simulink model "PMSM_foc_mod"  (R2020a)
settings: Solver=ode45  StartTime=0.0  StopTime=.5  MaxStep=1e-3  RelTol=1e-3
InitFcn:
  | %Rs = 2.98;
  | %phi_mg = .125;
  | %Jm = .47/10000;
  | %Bv = 1.1/10000;
  | %Zp = 2;
  | %Ld = 7/1000;
  | %Lq = 7/1000;
  | %Tl = 0;
  | 
  | Rs = 4.3;
  | phi_mg = .272;
  | Jm = .000179;
  | Bv = 1.1/10000;
  | Zp = 4;
  | Ld = 67e-3;
  | Lq = 67e-3;
  | Tl = 0;
  | 
  | Vdc = 220*2*sqrt(2);
libraries: powerlib x17, simulink x6, dspsigops x3, powerlib_meascontrol x3
settings Model: Creator=TELE  LastModifiedBy=TELE
settings DataIOCC: ReturnWorkspaceOutputs=off
settings DebuggingCC: ArithmeticOperatorsInVariantConditions=warning
settings SFSimCC: SimUseLocalCustomCode=off  CustomCodeUndefinedFunction=UseInterfaceOnly
settings RTWCC: RTWUseLocalCustomCode=off

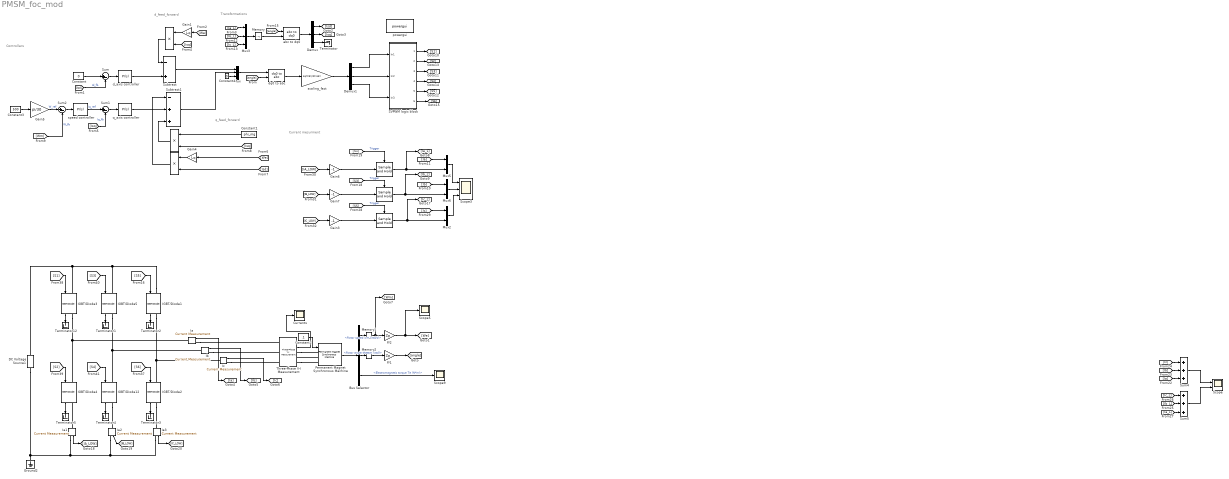
== system PMSM_foc_mod ==
  note: Controllers
  note: Transformations
  note: Current mesurment
  note: d_feed_forward
  note: q_feed_forward
  "  " : dspsigops/Sample and Hold  trig=Rising edge  initCond=0  latchinput=off
  "     " : dspsigops/Sample and Hold  trig=Rising edge  initCond=0  latchinput=off
  "         " : Product
  "           " : Product
  "                         " : Product
  "                                " : dspsigops/Sample and Hold  trig=Rising edge  initCond=0  latchinput=off
  Bus Selector : BusSelector  OutputSignals=Rotor speed wm (rad/s),Rotor angle thetam (rad),Electromagnetic torque Te (N*m)
  Constant : Constant  Value=0
  Constant1 : Constant  Value=phi_mg
  Constant2 : Constant  Value=.1
  Constant3 : Constant  Value=500
  Constant4 : Constant  Value=0
  Currents : Scope
  DC Voltage Source1 : powerlib/Electrical Sources/DC Voltage Source  Amplitude=Vdc  Measurements=None
  Demux : Demux  Outputs=3
  Demux1 : Demux  Outputs=3
  Gain1 : Gain  Gain=Lq
  Gain3 : Gain  Gain=-1
  Gain4 : Gain  Gain=Lq
  Gain5 : Gain  Gain=pi/30
  Gain6 : Gain  Gain=-1
  Gain7 : Gain  Gain=-1
  Ground2 : powerlib/Elements/Ground  LConnTagsString=a
  IGBT/Diode{1..5,12} (6 alike) : powerlib/Power Electronics/IGBT//Diode  Ron=1e-3  Rs=1e5  Cs=inf  Measurements=on
  Ia{,1..3} (4 alike) : powerlib/Measurements/Current Measurement  PhasorSimulation=off  OutputType=Complex  PSBequivalent=0
  Ib : powerlib/Measurements/Current Measurement  PhasorSimulation=off  OutputType=Complex  PSBequivalent=0
  Ic : powerlib/Measurements/Current Measurement  PhasorSimulation=off  OutputType=Complex  PSBequivalent=0
  Memory : Memory
  Memory1 : Memory
  Memory2 : Memory
  Mux : Mux  Inputs=3
  Mux2 : Mux  Inputs=2
  Mux3 : Mux  Inputs=3
  Mux5 : Mux  Inputs=2
  Mux6 : Mux  Inputs=2
  P/1 : Gain  Gain=Zp
  P/2 : Gain  Gain=Zp
  Permanent Magnet Synchronous Machine : powerlib/Machines/Permanent Magnet Synchronous Machine  NbPhases=3  FluxDistribution=Sinusoidal  RotorType=Round  MechanicalLoad=Torque Tm  PresetModel=No  ShowDetailedParameters=on  MeasurementBus=off  Resistance=Rs  Inductance=8.5e-3  dqInductances=[8.5e-3,8.5e-3]  La=Ld  MachineConstant=Flux linkage established by magnets (V.s)  Flux=phi_mg  VoltageCst=197.3414  TorqueCst=1.632  Flat=120  Mechanical=[Jm Bv Zp 0]  PolePairs=4  InitialConditions=[0,0, 0,0]  InitialConditions5ph=[0 0 0 0 0 0]  RefAngle=90 degrees behind phase A axis (modified Park)  IterativeDiscreteModel=Trapezoidal non iterative  TsBlock=-1  TsPowergui=0
  SVPWM logic block : Subsystem
  Scope : Scope  NumInputPorts=2
  Scope3 : Scope  NumInputPorts=3
  Scope5 : Scope
  Scope9 : Scope
  Subtract : Sum  Inputs=-+
  Subtract1 : Sum  Inputs=-++
  Sum : Sum  Inputs=|+-
  Sum1 : Sum  Inputs=|+-
  Sum2 : Sum  Inputs=|+-
  Sum4 : Sum  Inputs=+++
  Sum5 : Sum  Inputs=+++
  Terminator{,1..5,12} (7 alike) : Terminator
  Three-Phase V-I Measurement : powerlib/Measurements/Three-Phase V-I Measurement  VoltageMeasurement=phase-to-ground  SetLabelV=off  LabelV=Vabc  Vpu=off  VpuLL=off  CurrentMeasurement=yes  SetLabelI=off  LabelI=Iabc  Ipu=off  Pbase=100e6  Vbase=500e3  OutputType=Complex  PhasorSimulation=off  PSBequivalent=0
  abc to dq0 : powerlib_meascontrol/Transformations/abc to dq0  Alignment=90 degrees behind phase A axis
  d_axis controller : simulink/Continuous/PID Controller  Controller=PI  Form=Parallel  TimeDomain=Continuous-time  UseExternalTs=off  SampleTime=-1  IntegratorMethod=Forward Euler  FilterMethod=Forward Euler  ControllerParametersSource=internal  P=190.322068059803  I=236063.180042371  D=0  UseFilter=on  N=100  TunerSelectOption=Transfer Function Based (PID Tuner App)  InitialConditionSource=internal  InitialConditionForIntegrator=0  InitialConditionForFilter=0  DifferentiatorICPrevScaledInput=0  ExternalReset=none  TrackingMode=off  Kt=1  LimitOutput=off  UpperSaturationLimit=inf  LowerSaturationLimit=-inf  LinearizeAsGain=on  AntiWindupMode=none  Kb=1  POutMin=[]  POutMax=[]  IOutMin=[]  IOutMax=[]  DOutMin=[]  DOutMax=[]  NOutMin=[]  NOutMax=[]  SumOutMin=[]  SumOutMax=[]  SaturationOutMin=[]  SaturationOutMax=[]  PParamMin=[]  PParamMax=[]  IParamMin=[]  IParamMax=[]  DParamMin=[]  DParamMax=[]  NParamMin=[]  NParamMax=[]  KbParamMin=[]  KbParamMax=[]  KtParamMin=[]  KtParamMax=[]  KbOutMin=[]  KbOutMax=[]  KtOutMin=[]  KtOutMax=[]  IntegratorOutMin=[]  IntegratorOutMax=[]  FilterOutMin=[]  FilterOutMax=[]  SumI1OutMin=[]  SumI1OutMax=[]  SumI2OutMin=[]  SumI2OutMax=[]  SumI3OutMin=[]  SumI3OutMax=[]  SumI4OutMin=[]  SumI4OutMax=[]  SumDOutMin=[]  SumDOutMax=[]  DifferentiatorOutMin=[]  DifferentiatorOutMax=[]  FilterDiffOutCoefMin=[]  FilterDiffOutCoefMax=[]  ReciprocalOutMin=[]  ReciprocalOutMax=[]  SumDenOutMin=[]  SumDenOutMax=[]  SumNumOutMin=[]  SumNumOutMax=[]  DivideOutMin=[]  DivideOutMax=[]  UdiffTsProdOutMin=[]  UdiffTsProdOutMax=[]  NTsProdOutMin=[]  NTsProdOutMax=[]  UintegralTsProdOutMin=[]  UintegralTsProdOutMax=[]  UngainTsProdOutMin=[]  UngainTsProdOutMax=[]  IntegratorContinuousStateAttributes=''  IntegratorStateMustResolveToSignalObject=off  IntegratorRTWStateStorageClass=Auto  FilterContinuousStateAttributes=''  FilterStateMustResolveToSignalObject=off  FilterRTWStateStorageClass=Auto  ParallelPVariant=InternalParameters  IdealPVariant=Disabled  IVariant=InternalParameters  DVariant=Disabled  IntegratorVariant=Continuous  SatVariant=Disabled  AWVariant=Passthrough  PCopyVariant=Disabled  TRVariant=Disabled  FdbkBlocksVariant=Forward  IdealPFdbkVariant=Disabled  SatFdbkVariant=Disabled  DerivativeFilterVariant=Disabled  NVariant=Disabled  NCopyVariant=Disabled_SignalSpec  FilterICVariant=Disabled  IntegratorICVariant=InternalICs  ExternalResetVariant=Disabled  TRSumVariant=Passthrough  SumFdbkVariant=Disabled  SumVariant=Sum_PI  TsampFilterVariant=InternalTs  TsampNgainVariant=Passthrough  TsampIntegralVariant=Passthrough
  dq0 to abc : powerlib_meascontrol/Transformations/dq0 to abc  Alignment=90 degrees behind phase A axis
  powergui : powerlib/powergui  Priority=1  SimulationMode=Continuous  SampleTime=50e-6  frequency=60  Iterations=50  frequencyindice=0  Pbase=100e6  ErrMax=1e-4  UnitsV=kV  UnitsW=MW  buscounter=0  FunctionMessages=off  echomessages=off  EnableUseOfTLC=off  CurrentSourceSwitches=off  DisableSnubberDevices=off  DisableRonSwitches=off  DisableVfSwitches=off  DisplayEquations=off  AutomaticDiscreteSolvers=off  SolverType=Tustin/Backward Euler (TBE)  Interpol=off  ExternalGateDelay=off  methode=off  Ts=100  x0status=blocks  SPID=on  SwTol=0  HookPort=off  NonlinearTolerance=1e-4  nMaxIteration=100  ContinueOnMaxIteration=off  RestoreLinks=warning  ResistiveCurrentMeasurement=off  Frange=[0:2:500]  Ylog=off  Xlog=on  ShowGrid=off  save=off  variable=ZData  structure=0  ZoomFFT=off  StartTime=0.0  cycles=1  DisplayStyle=1  fundamental=60  FreqAxis=off  MaxFrequency=1000  frequencyindicesteady=1  RmsSteady=1  display=off
  q_axis controller : simulink/Continuous/PID Controller  Controller=PI  Form=Parallel  TimeDomain=Continuous-time  UseExternalTs=off  SampleTime=-1  IntegratorMethod=Forward Euler  FilterMethod=Forward Euler  ControllerParametersSource=internal  P=190.322068059803  I=236063.180042371  D=0  UseFilter=on  N=100  TunerSelectOption=Transfer Function Based (PID Tuner App)  InitialConditionSource=internal  InitialConditionForIntegrator=0  InitialConditionForFilter=0  DifferentiatorICPrevScaledInput=0  ExternalReset=none  TrackingMode=off  Kt=1  LimitOutput=off  UpperSaturationLimit=inf  LowerSaturationLimit=-inf  LinearizeAsGain=on  AntiWindupMode=none  Kb=1  POutMin=[]  POutMax=[]  IOutMin=[]  IOutMax=[]  DOutMin=[]  DOutMax=[]  NOutMin=[]  NOutMax=[]  SumOutMin=[]  SumOutMax=[]  SaturationOutMin=[]  SaturationOutMax=[]  PParamMin=[]  PParamMax=[]  IParamMin=[]  IParamMax=[]  DParamMin=[]  DParamMax=[]  NParamMin=[]  NParamMax=[]  KbParamMin=[]  KbParamMax=[]  KtParamMin=[]  KtParamMax=[]  KbOutMin=[]  KbOutMax=[]  KtOutMin=[]  KtOutMax=[]  IntegratorOutMin=[]  IntegratorOutMax=[]  FilterOutMin=[]  FilterOutMax=[]  SumI1OutMin=[]  SumI1OutMax=[]  SumI2OutMin=[]  SumI2OutMax=[]  SumI3OutMin=[]  SumI3OutMax=[]  SumI4OutMin=[]  SumI4OutMax=[]  SumDOutMin=[]  SumDOutMax=[]  DifferentiatorOutMin=[]  DifferentiatorOutMax=[]  FilterDiffOutCoefMin=[]  FilterDiffOutCoefMax=[]  ReciprocalOutMin=[]  ReciprocalOutMax=[]  SumDenOutMin=[]  SumDenOutMax=[]  SumNumOutMin=[]  SumNumOutMax=[]  DivideOutMin=[]  DivideOutMax=[]  UdiffTsProdOutMin=[]  UdiffTsProdOutMax=[]  NTsProdOutMin=[]  NTsProdOutMax=[]  UintegralTsProdOutMin=[]  UintegralTsProdOutMax=[]  UngainTsProdOutMin=[]  UngainTsProdOutMax=[]  IntegratorContinuousStateAttributes=''  IntegratorStateMustResolveToSignalObject=off  IntegratorRTWStateStorageClass=Auto  FilterContinuousStateAttributes=''  FilterStateMustResolveToSignalObject=off  FilterRTWStateStorageClass=Auto  ParallelPVariant=InternalParameters  IdealPVariant=Disabled  IVariant=InternalParameters  DVariant=Disabled  IntegratorVariant=Continuous  SatVariant=Disabled  AWVariant=Passthrough  PCopyVariant=Disabled  TRVariant=Disabled  FdbkBlocksVariant=Forward  IdealPFdbkVariant=Disabled  SatFdbkVariant=Disabled  DerivativeFilterVariant=Disabled  NVariant=Disabled  NCopyVariant=Disabled_SignalSpec  FilterICVariant=Disabled  IntegratorICVariant=InternalICs  ExternalResetVariant=Disabled  TRSumVariant=Passthrough  SumFdbkVariant=Disabled  SumVariant=Sum_PI  TsampFilterVariant=InternalTs  TsampNgainVariant=Passthrough  TsampIntegralVariant=Passthrough
  scaling_fact : Gain  Gain=sqrt(3)/(2*Vdc)
  speed controller : simulink/Continuous/PID Controller  Controller=PI  Form=Parallel  TimeDomain=Continuous-time  UseExternalTs=off  SampleTime=-1  IntegratorMethod=Forward Euler  FilterMethod=Forward Euler  ControllerParametersSource=internal  P=0.003810758400944  I=0.0139378856974398  D=0  UseFilter=on  N=100  TunerSelectOption=Transfer Function Based (PID Tuner App)  InitialConditionSource=internal  InitialConditionForIntegrator=0  InitialConditionForFilter=0  DifferentiatorICPrevScaledInput=0  ExternalReset=none  TrackingMode=off  Kt=1  LimitOutput=off  UpperSaturationLimit=inf  LowerSaturationLimit=-inf  LinearizeAsGain=on  AntiWindupMode=none  Kb=1  POutMin=[]  POutMax=[]  IOutMin=[]  IOutMax=[]  DOutMin=[]  DOutMax=[]  NOutMin=[]  NOutMax=[]  SumOutMin=[]  SumOutMax=[]  SaturationOutMin=[]  SaturationOutMax=[]  PParamMin=[]  PParamMax=[]  IParamMin=[]  IParamMax=[]  DParamMin=[]  DParamMax=[]  NParamMin=[]  NParamMax=[]  KbParamMin=[]  KbParamMax=[]  KtParamMin=[]  KtParamMax=[]  KbOutMin=[]  KbOutMax=[]  KtOutMin=[]  KtOutMax=[]  IntegratorOutMin=[]  IntegratorOutMax=[]  FilterOutMin=[]  FilterOutMax=[]  SumI1OutMin=[]  SumI1OutMax=[]  SumI2OutMin=[]  SumI2OutMax=[]  SumI3OutMin=[]  SumI3OutMax=[]  SumI4OutMin=[]  SumI4OutMax=[]  SumDOutMin=[]  SumDOutMax=[]  DifferentiatorOutMin=[]  DifferentiatorOutMax=[]  FilterDiffOutCoefMin=[]  FilterDiffOutCoefMax=[]  ReciprocalOutMin=[]  ReciprocalOutMax=[]  SumDenOutMin=[]  SumDenOutMax=[]  SumNumOutMin=[]  SumNumOutMax=[]  DivideOutMin=[]  DivideOutMax=[]  UdiffTsProdOutMin=[]  UdiffTsProdOutMax=[]  NTsProdOutMin=[]  NTsProdOutMax=[]  UintegralTsProdOutMin=[]  UintegralTsProdOutMax=[]  UngainTsProdOutMin=[]  UngainTsProdOutMax=[]  IntegratorContinuousStateAttributes=''  IntegratorStateMustResolveToSignalObject=off  IntegratorRTWStateStorageClass=Auto  FilterContinuousStateAttributes=''  FilterStateMustResolveToSignalObject=off  FilterRTWStateStorageClass=Auto  ParallelPVariant=InternalParameters  IdealPVariant=Disabled  IVariant=InternalParameters  DVariant=Disabled  IntegratorVariant=Continuous  SatVariant=Disabled  AWVariant=Passthrough  PCopyVariant=Disabled  TRVariant=Disabled  FdbkBlocksVariant=Forward  IdealPFdbkVariant=Disabled  SatFdbkVariant=Disabled  DerivativeFilterVariant=Disabled  NVariant=Disabled  NCopyVariant=Disabled_SignalSpec  FilterICVariant=Disabled  IntegratorICVariant=InternalICs  ExternalResetVariant=Disabled  TRSumVariant=Passthrough  SumFdbkVariant=Disabled  SumVariant=Sum_PI  TsampFilterVariant=InternalTs  TsampNgainVariant=Passthrough  TsampIntegralVariant=Passthrough
  wires:
  Ia/1 -> [Ia]
  Bus Selector/3 -> Scope9/1  "<Electromagnetic torque Te (N*m)>"
  P/2/1 -> Scope5/1, [We]
  Demux1/3 -> SVPWM logic block/3(In3)
  Demux1/2 -> SVPWM logic block/2(In2)
  Demux1/1 -> SVPWM logic block/1(In1)
  scaling_fact/1 -> Demux1/1
  SVPWM logic block/5(5) -> [S5]
  [S4] -> IGBT/Diode12/1
  IGBT/Diode12/1 -> Terminator4/1
  [S5] -> IGBT/Diode1/1
  [S2] -> IGBT/Diode4/1
  SVPWM logic block/3(3) -> [S3]
  [S3] -> IGBT/Diode5/1
  IGBT/Diode2/1 -> Terminator3/1
  IGBT/Diode3/1 -> Terminator12/1
  SVPWM logic block/1(1) -> [S1]
  SVPWM logic block/4(4) -> [S4]
  IGBT/Diode5/1 -> Terminator1/1
  [S1] -> IGBT/Diode3/1
  IGBT/Diode4/1 -> Terminator5/1
  SVPWM logic block/2(2) -> [S2]
  IGBT/Diode1/1 -> Terminator2/1
  [S6] -> IGBT/Diode2/1
  SVPWM logic block/6(6) -> [S6]
  Demux/3 -> Terminator/1
  Demux/2 -> [Isq]
  Demux/1 -> [Isd]
  abc to dq0/1 -> Demux/1
  [angle] -> abc to dq0/2
  Ic/1 -> [Ic]
  Ib/1 -> [Ib]
  [angle] -> dq0 to abc/2
  P/1/1 -> [angle]
  Bus Selector/2 -> Memory2/1  "<Rotor angle thetam (rad)>"
  Mux/1 -> dq0 to abc/1
  Memory1/1 -> [Wm], P/2/1
  Permanent Magnet Synchronous Machine/1 -> Bus Selector/1
  "                         "/1 -> Subtract1/3
  Constant1/1 -> "                         "/1
  [Isq] -> "                         "/2
  q_axis controller/1 -> Subtract1/2
  Sum1/1 -> q_axis controller/1
  [We] -> Gain4/1
  Gain4/1 -> "         "/1
  [Isd] -> "         "/2
  "         "/1 -> Subtract1/1
  Subtract1/1 -> Mux/2
  Subtract/1 -> Mux/1
  "           "/1 -> Subtract/1
  [Isq] -> "           "/2
  Gain1/1 -> "           "/1
  [We] -> Gain1/1
  Sum/1 -> d_axis controller/1
  d_axis controller/1 -> Subtract/2
  speed controller/1 -> Sum1/1  "Iq_ref"
  Sum2/1 -> speed controller/1
  Constant3/1 -> Gain5/1
  Constant2/1 -> Permanent Magnet Synchronous Machine/1
  Constant4/1 -> Mux/3
  Three-Phase V-I Measurement/2 -> Currents/1
  Gain5/1 -> Sum2/1  "W_ref"
  Gain6/1 -> "  "/1
  Gain7/1 -> "     "/1
  "     "/1 -> [Ib_L], Mux6/2
  "  "/1 -> [Ia_L], Mux5/2
  [S3] -> "     "/Trigger  "Trigger"
  Mux5/1 -> Scope3/1
  Mux6/1 -> Scope3/2
  [Ib] -> Mux6/1
  [Ia] -> Mux5/1
  [S1] -> "  "/Trigger  "Trigger"
  Mux3/1 -> Memory/1
  dq0 to abc/1 -> scaling_fact/1
  Constant/1 -> Sum/1
  [Isd] -> Sum/2  "Id_fb"
  [Wm] -> Sum2/2  "W_fb"
  [Isq] -> Sum1/2  "Iq_fb"
  Memory/1 -> abc to dq0/1
  [Ia_L] -> Mux3/1
  [Ic_L] -> Mux3/3
  [Ib_L] -> Mux3/2
  Sum4/1 -> Scope/1
  [Ib] -> Sum4/2
  [Ic] -> Sum4/1
  [Ia] -> Sum4/3
  [Ic_L] -> Sum5/1
  [Ib_L] -> Sum5/2
  [Ia_L] -> Sum5/3
  Sum5/1 -> Scope/2
  [S5] -> "                                "/Trigger  "Trigger"
  Gain3/1 -> "                                "/1
  "                                "/1 -> Mux2/2, [Ic_L]
  [Ic] -> Mux2/1
  Mux2/1 -> Scope3/3
  Bus Selector/1 -> Memory1/1  "<Rotor speed wm (rad/s)>"
  Memory2/1 -> P/1/1
  Ia1/1 -> [IA_LOW]
  Ia2/1 -> [IB_LOW]
  Ia3/1 -> [IC_LOW]
  [IA_LOW] -> Gain6/1
  [IB_LOW] -> Gain7/1
  [IC_LOW] -> Gain3/1
  connections:
  IGBT/Diode1/LConn1 -- IGBT/Diode3/LConn1 -- DC Voltage Source1/RConn1 -- IGBT/Diode5/LConn1
  DC Voltage Source1/LConn1 -- Ground2/LConn1 -- Ia1/RConn1 -- Ia3/RConn1 -- Ia2/RConn1
  IGBT/Diode5/RConn1 -- IGBT/Diode12/LConn1 -- Ib/LConn1
  IGBT/Diode3/RConn1 -- IGBT/Diode4/LConn1 -- Ia/LConn1
  IGBT/Diode1/RConn1 -- Ic/LConn1 -- IGBT/Diode2/LConn1
  Three-Phase V-I Measurement/RConn3 -- Permanent Magnet Synchronous Machine/LConn3
  Permanent Magnet Synchronous Machine/LConn2 -- Three-Phase V-I Measurement/RConn2
  Three-Phase V-I Measurement/RConn1 -- Permanent Magnet Synchronous Machine/LConn1
  Ic/RConn1 -- Three-Phase V-I Measurement/LConn3
  Ib/RConn1 -- Three-Phase V-I Measurement/LConn2
  Ia/RConn1 -- Three-Phase V-I Measurement/LConn1
  Ia1/LConn1 -- IGBT/Diode4/RConn1
  IGBT/Diode12/RConn1 -- Ia2/LConn1
  IGBT/Diode2/RConn1 -- Ia3/LConn1

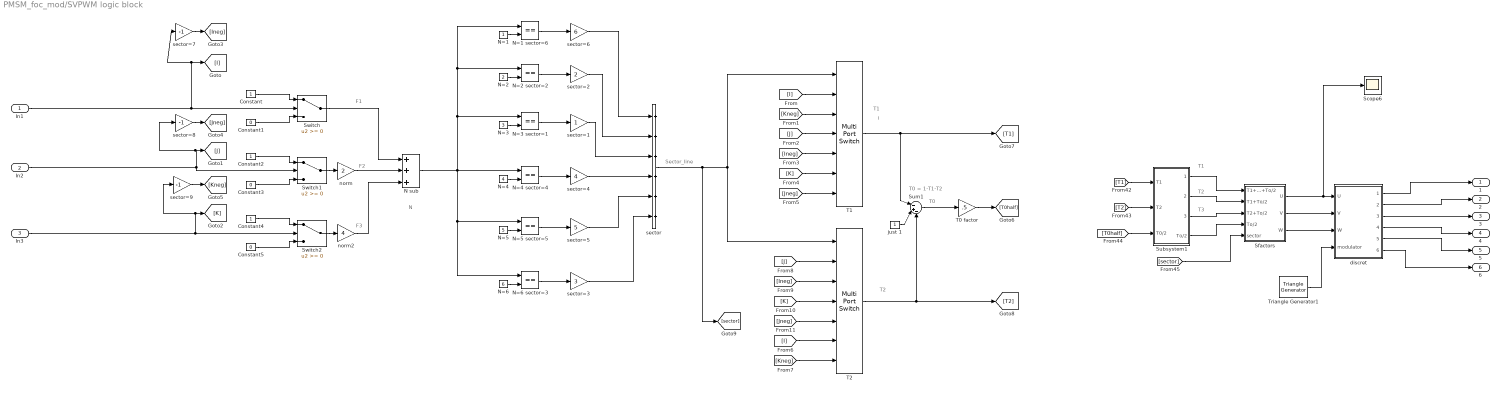
== system PMSM_foc_mod/SVPWM logic block ==
  note: N
  note: Sector_line
  note: i
  note: T1
  note: T2
  note: T0 = 1-T1-T2
  note: T0
  note: F1
  note: F2
  note: F3
  note: T1
  note: T2
  note: T3
  In1 : Inport
  In2 : Inport  Port=2
  In3 : Inport  Port=3
  Constant : Constant
  Constant1 : Constant  Value=0
  Constant2 : Constant
  Constant3 : Constant  Value=0
  Constant4 : Constant
  Constant5 : Constant  Value=0
  N sub : Sum  Inputs=+++
  N=1 : Constant
  N=1 sector=6 : RelationalOperator  Operator===  OutDataTypeStr=boolean  RndMeth=Nearest
  N=2 : Constant  Value=2
  N=2 sector=2 : RelationalOperator  Operator===  OutDataTypeStr=boolean  RndMeth=Nearest
  N=3 : Constant  Value=3
  N=3 sector=1 : RelationalOperator  Operator===  OutDataTypeStr=boolean  RndMeth=Nearest
  N=4 : Constant  Value=4
  N=4 sector=4 : RelationalOperator  Operator===  OutDataTypeStr=boolean  RndMeth=Nearest
  N=5 : Constant  Value=5
  N=5 sector=5 : RelationalOperator  Operator===  OutDataTypeStr=boolean  RndMeth=Nearest
  N=6 : Constant  Value=6
  N=6 sector=3 : RelationalOperator  Operator===  OutDataTypeStr=boolean  RndMeth=Nearest
  Scope6 : Scope
  Sfactors : Subsystem
  Subsystem1 : Subsystem
  Sum1 : Sum  Inputs=|-+-
  Switch : Switch
  Switch1 : Switch
  Switch2 : Switch
  T0 factor : Gain  Gain=.5
  T1 : MultiPortSwitch  DataPortOrder=Specify indices  Inputs=4  DataPortIndices={1,2,3,4,5,6}  DiagnosticForDefault=None
  T2 : MultiPortSwitch  DataPortOrder=Specify indices  Inputs=4  DataPortIndices={1,2,3,4,5,6}  DiagnosticForDefault=None
  Triangle Generator1 : powerlib_meascontrol/Pulse & Signal Generators/Triangle Generator  Freq=40e3  Phase=180  Ts=0
  discret : Subsystem
  just 1 : Constant
  norm : Gain  Gain=2
  norm2 : Gain  Gain=4
  sector : Sum  Inputs=++++++
  sector=1 : Gain
  sector=2 : Gain  Gain=2
  sector=3 : Gain  Gain=3
  sector=4 : Gain  Gain=4
  sector=5 : Gain  Gain=5
  sector=6 : Gain  Gain=6
  sector=7 : Gain  Gain=-1
  sector=8 : Gain  Gain=-1
  sector=9 : Gain  Gain=-1
  1 : Outport  VectorParamsAs1DForOutWhenUnconnected=off
  2 : Outport  Port=2  VectorParamsAs1DForOutWhenUnconnected=off
  3 : Outport  Port=3  VectorParamsAs1DForOutWhenUnconnected=off
  4 : Outport  Port=4  VectorParamsAs1DForOutWhenUnconnected=off
  5 : Outport  Port=5  VectorParamsAs1DForOutWhenUnconnected=off
  6 : Outport  Port=6  VectorParamsAs1DForOutWhenUnconnected=off
  wires:
  discret/6(6) -> 6/1
  discret/5(5) -> 5/1
  Sfactors/1(U) -> discret/1(U), Scope6/1
  Subsystem1/3(T2+To/2) -> Sfactors/3(T2+To/2)
  [sector] -> Sfactors/5("sector ")
  Subsystem1/4(To/2) -> Sfactors/4(To/2)
  Sfactors/2(V) -> discret/2(V)
  [T2] -> Subsystem1/2(T2)
  T2/1 -> [T2], Sum1/3
  discret/1(1) -> 1/1
  [T0half] -> Subsystem1/3(T0/2)
  [T1] -> Subsystem1/1(T1)
  Subsystem1/1(T1+T2+To/2) -> Sfactors/1(T1+T2+To/2)
  discret/4(4) -> 4/1
  Subsystem1/2(T1+To/2) -> Sfactors/2(T1+To/2)
  discret/3(3) -> 3/1
  discret/2(2) -> 2/1
  Triangle Generator1/1 -> discret/4(modulator)
  Sfactors/3(W) -> discret/3(W)
  [Ineg] -> T2/3
  norm/1 -> N sub/2
  [Jneg] -> T2/5
  [Kneg] -> T1/3
  just 1/1 -> Sum1/2
  sector=9/1 -> [Kneg]
  T1/1 -> Sum1/1, [T1]
  [K] -> T2/4
  [I] -> T2/6
  [J] -> T1/4
  [K] -> T1/6
  [J] -> T2/2
  [Jneg] -> T1/7
  norm2/1 -> N sub/3
  sector=7/1 -> [Ineg]
  [Ineg] -> T1/5
  sector/1 -> T1/1, T2/1, [sector]
  T0 factor/1 -> [T0half]
  Sum1/1 -> T0 factor/1
  sector=8/1 -> [Jneg]
  [Kneg] -> T2/7
  [I] -> T1/2
  Constant5/1 -> Switch2/3
  In3/1 -> [K], sector=9/1, Switch2/2
  sector=6/1 -> sector/1
  N=1 sector=6/1 -> sector=6/1
  sector=3/1 -> sector/6
  Switch1/1 -> norm/1
  sector=1/1 -> sector/3
  N=4 sector=4/1 -> sector=4/1
  sector=5/1 -> sector/5
  sector=4/1 -> sector/4
  N=2 sector=2/1 -> sector=2/1
  sector=2/1 -> sector/2
  N=2/1 -> N=2 sector=2/2
  Switch2/1 -> norm2/1
  N=5 sector=5/1 -> sector=5/1
  N=4/1 -> N=4 sector=4/2
  In2/1 -> sector=8/1, [J], Switch1/2
  Switch/1 -> N sub/1
  Constant4/1 -> Switch2/1
  N=3/1 -> N=3 sector=1/2
  N=3 sector=1/1 -> sector=1/1
  N sub/1 -> N=1 sector=6/1, N=2 sector=2/1, N=3 sector=1/1, N=4 sector=4/1, N=5 sector=5/1, N=6 sector=3/1
  N=5/1 -> N=5 sector=5/2
  N=6 sector=3/1 -> sector=3/1
  N=6/1 -> N=6 sector=3/2
  N=1/1 -> N=1 sector=6/2
  Constant3/1 -> Switch1/3
  Constant/1 -> Switch/1
  Constant2/1 -> Switch1/1
  In1/1 -> [I], sector=7/1, Switch/2
  Constant1/1 -> Switch/3

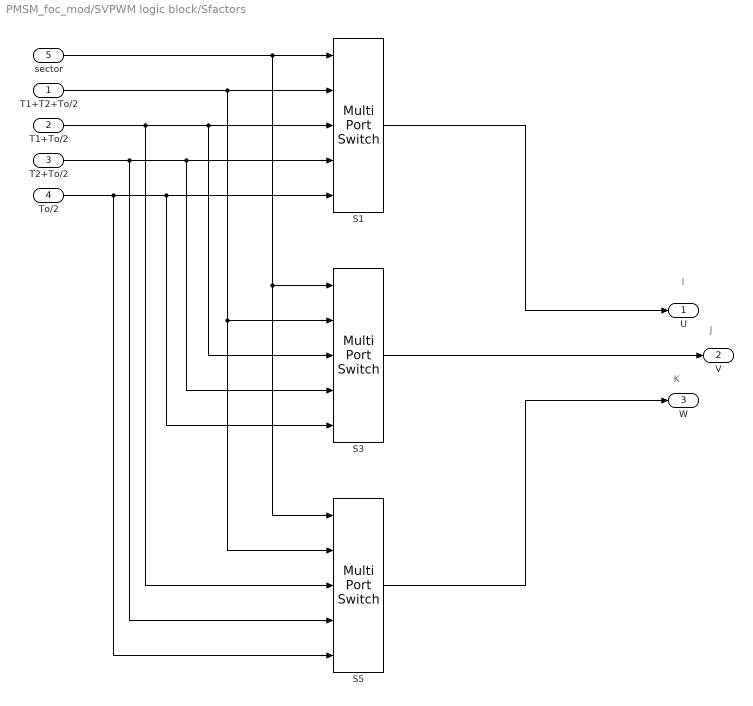
== system PMSM_foc_mod/SVPWM logic block/Sfactors ==
  note: I
  note: J
  note: K
  T1+T2+To/2 : Inport
  T1+To/2 : Inport  Port=2
  T2+To/2 : Inport  Port=3
  To/2 : Inport  Port=4
  "sector " : Inport  Port=5
  S1 : MultiPortSwitch  DataPortOrder=Specify indices  Inputs=4  DataPortIndices={[1,6],2,5,[3,4]}  DiagnosticForDefault=None
  S3 : MultiPortSwitch  DataPortOrder=Specify indices  Inputs=4  DataPortIndices={[2,3],4,1,[5,6]}  DiagnosticForDefault=None
  S5 : MultiPortSwitch  DataPortOrder=Specify indices  Inputs=4  DataPortIndices={[4,5],6,3,[1,2]}  DiagnosticForDefault=None
  U : Outport  VectorParamsAs1DForOutWhenUnconnected=off
  V : Outport  Port=2  VectorParamsAs1DForOutWhenUnconnected=off
  W : Outport  Port=3  VectorParamsAs1DForOutWhenUnconnected=off
  wires:
  "sector "/1 -> S1/1, S5/1, S3/1
  S3/1 -> V/1
  T2+To/2/1 -> S3/4, S1/4, S5/4
  S5/1 -> W/1
  T1+To/2/1 -> S3/3, S1/3, S5/3
  T1+T2+To/2/1 -> S1/2, S5/2, S3/2
  To/2/1 -> S3/5, S1/5, S5/5
  S1/1 -> U/1

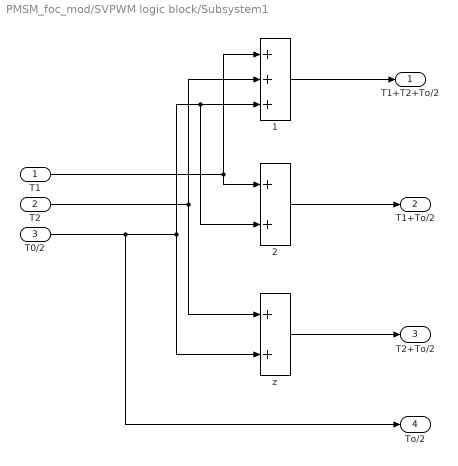
== system PMSM_foc_mod/SVPWM logic block/Subsystem1 ==
  T1 : Inport
  T2 : Inport  Port=2
  T0/2 : Inport  Port=3
  1 : Sum  Inputs=+++
  2 : Sum
  z : Sum
  T1+T2+To/2 : Outport  VectorParamsAs1DForOutWhenUnconnected=off
  T1+To/2 : Outport  Port=2  VectorParamsAs1DForOutWhenUnconnected=off
  T2+To/2 : Outport  Port=3  VectorParamsAs1DForOutWhenUnconnected=off
  To/2 : Outport  Port=4  VectorParamsAs1DForOutWhenUnconnected=off
  wires:
  z/1 -> T2+To/2/1
  T2/1 -> 1/2, z/1
  1/1 -> T1+T2+To/2/1
  2/1 -> T1+To/2/1
  T0/2/1 -> To/2/1, 2/2, 1/3, z/2
  T1/1 -> 1/1, 2/1

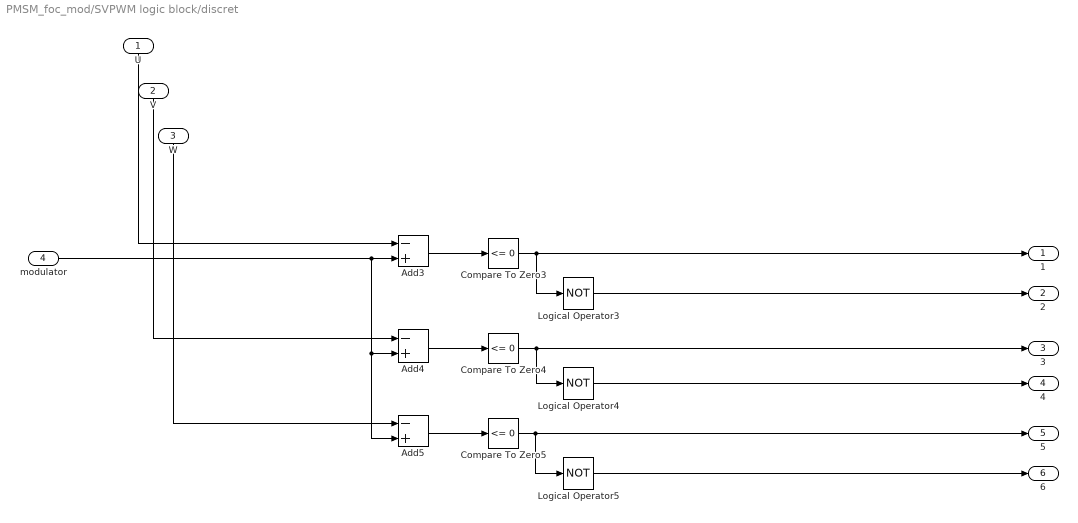
== system PMSM_foc_mod/SVPWM logic block/discret ==
  U : Inport
  V : Inport  Port=2
  W : Inport  Port=3
  modulator : Inport  Port=4
  Add3 : Sum  Inputs=-+
  Add4 : Sum  Inputs=-+
  Add5 : Sum  Inputs=-+
  Compare To Zero3 : simulink/Logic and Bit Operations/Compare To Zero  relop=<=  OutDataTypeStr=boolean
  Compare To Zero4 : simulink/Logic and Bit Operations/Compare To Zero  relop=<=  OutDataTypeStr=boolean
  Compare To Zero5 : simulink/Logic and Bit Operations/Compare To Zero  relop=<=  OutDataTypeStr=boolean
  Logical Operator3 : Logic  Operator=NOT  AllPortsSameDT=off  OutDataTypeStr=boolean
  Logical Operator4 : Logic  Operator=NOT  AllPortsSameDT=off  OutDataTypeStr=boolean
  Logical Operator5 : Logic  Operator=NOT  AllPortsSameDT=off  OutDataTypeStr=boolean
  1 : Outport  VectorParamsAs1DForOutWhenUnconnected=off
  2 : Outport  Port=2  VectorParamsAs1DForOutWhenUnconnected=off
  3 : Outport  Port=3  VectorParamsAs1DForOutWhenUnconnected=off
  4 : Outport  Port=4  VectorParamsAs1DForOutWhenUnconnected=off
  5 : Outport  Port=5  VectorParamsAs1DForOutWhenUnconnected=off
  6 : Outport  Port=6  VectorParamsAs1DForOutWhenUnconnected=off
  wires:
  modulator/1 -> Add4/2, Add5/2, Add3/2
  Add4/1 -> Compare To Zero4/1
  Add3/1 -> Compare To Zero3/1
  Add5/1 -> Compare To Zero5/1
  U/1 -> Add3/1
  W/1 -> Add5/1
  V/1 -> Add4/1
  Logical Operator5/1 -> 6/1
  Logical Operator4/1 -> 4/1
  Compare To Zero3/1 -> 1/1, Logical Operator3/1
  Logical Operator3/1 -> 2/1
  Compare To Zero5/1 -> 5/1, Logical Operator5/1
  Compare To Zero4/1 -> 3/1, Logical Operator4/1
